simulink model "verify_Average_mdl"  (R2016b)
settings: Solver=VariableStepDiscrete  StartTime=0  StopTime=24*3600  MaxStep=1  RelTol=1e-3  EnableMultiTasking=on
libraries: carnot x1
settings Model: Creator=drhf  LastModifiedBy=User
settings DataIOCC: SaveFormat=Array  SignalLoggingSaveFormat=ModelDataLogs
settings OptimizationCC: ExpressionDepthLimit=2147483647  LifeSpan=inf
settings DebuggingCC: UnderspecifiedInitializationDetection=Classic  MergeDetectMultiDrivingBlocksExec=none  SolverPrmCheckMsg=warning  FcnCallInpInsideContextMsg=warning  StateNameClashWarn=warning  SFUnexpectedBacktrackingDiag=warning  SFNoUnconditionalDefaultTransitionDiag=warning  SFExecutionAtInitializationDiag=none
settings HardwareCC: ProdBitPerPointer=32  ProdBitPerSizeT=32  ProdBitPerPtrDiffT=32  ProdLargestAtomicFloat=None  ProdIntDivRoundTo=Undefined  ProdEndianess=Unspecified  ProdWordSize=32  ProdHWDeviceType=32-bit Generic
settings ModelReferenceCC: PropagateSignalLabelsOutOfModel=off
settings GRTTargetCC: TargetLangStandard=C89/C90 (ANSI)  GeneratePreprocessorConditionals=Disable all  CombineOutputUpdateFcns=off  GRTInterface=on
settings ConfigComp: CovMetricSettings=dw  CovHtmlReporting=on  CovSaveCumulativeToWorkspaceVar=on  CovSaveSingleToWorkspaceVar=on  CovExternalEMLEnable=off

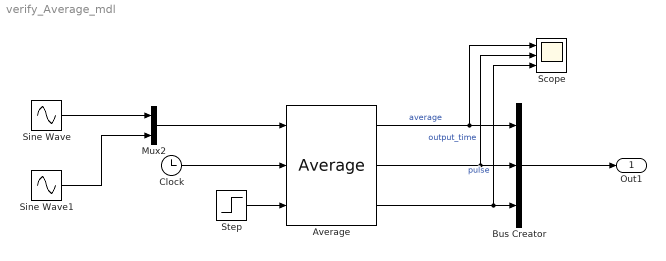
== system verify_Average_mdl ==
  Average : carnot/Toolbox/Average  time_intervall=1 h  offset_flag=on  enable_flag=on
  Bus Creator : BusCreator  Inputs=3
  Clock : Clock
  Mux2 : Mux  Inputs=2
  Scope : Scope  NumInputPorts=3
  Sine Wave : Sin  Frequency=2*pi/(24*3600)  SampleTime=0
  Sine Wave1 : Sin  Frequency=2*pi/(24*3600)  Phase=3*3600  SampleTime=0
  Step : Step  Time=3600  SampleTime=0
  Out1 : Outport
  wires:
  Bus Creator/1 -> Out1/1
  Average/2 -> Scope/2, Bus Creator/2  "output_time"
  Average/3 -> Scope/3, Bus Creator/3  "pulse"
  Average/1 -> Scope/1, Bus Creator/1  "average"
  Sine Wave/1 -> Mux2/1
  Sine Wave1/1 -> Mux2/2
  Mux2/1 -> Average/1
  Clock/1 -> Average/2
  Step/1 -> Average/3
